simulink model "OPTIM"  (Simulink 4.00)
settings: Solver=ode45  StartTime=0.0  StopTime=40  RelTol=1e-3
settings Model: BlockReductionOpt=off

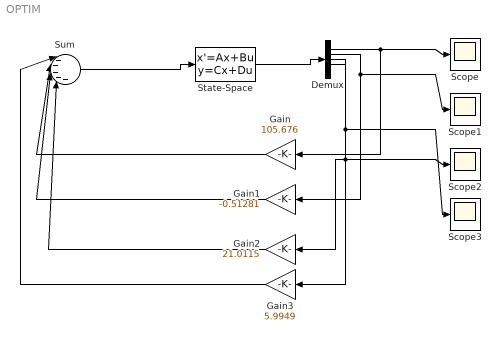
== system OPTIM ==
  Demux : Demux  Outputs=5  BusSelectionMode=off
  Gain : Gain  Orientation=left  Gain=105.676  Multiplication=Element-wise(K.*u)  SaturateOnIntegerOverflow=on
  Gain1 : Gain  Orientation=left  Gain=-0.51281  Multiplication=Element-wise(K.*u)  SaturateOnIntegerOverflow=on
  Gain2 : Gain  Orientation=left  Gain=21.0115  Multiplication=Element-wise(K.*u)  SaturateOnIntegerOverflow=on
  Gain3 : Gain  Orientation=left  Gain=5.9949  Multiplication=Element-wise(K.*u)  SaturateOnIntegerOverflow=on
  Scope{,1..3} (4 alike) : Scope
      Scope settings: TimeRange=auto  YMin=-10  YMax=10  SaveToWorkspace=off  SaveName=ScopeData  LimitDataPoints=on  MaxDataPoints=500000
      Scope1 settings: TimeRange=auto  YMin=-5  YMax=5  SaveToWorkspace=off  LimitDataPoints=on  MaxDataPoints=500000
      Scope2 settings: TimeRange=auto  YMin=-150  YMax=125  SaveToWorkspace=off  SaveName=ScopeData2  LimitDataPoints=on  MaxDataPoints=500000
      Scope3 settings: TimeRange=auto  YMin=-75  YMax=75  SaveToWorkspace=off  SaveName=ScopeData3  LimitDataPoints=on  MaxDataPoints=500000
  State-Space : StateSpace  A=[0 1 0 0 0; 0 -16 -9.8178 0 623.16; 0 0 0 1 0; -8.7478 0.15147 -3.2745 -0.02575 0; 0 -144740 0 0 -475]  B=[0 0 0 0 250]'  C="[1 0 0 0 0  ;0 1 0 0 0 ;0 0 1 0  0;0 0 0 1 0 ;0 0 0 0 1]"  D=[0 0 0 0 0]'  X0=[5 0 30 0 0]  Realization=auto  AbsoluteTolerance=auto
  Sum : Sum  Inputs=|-----  SaturateOnIntegerOverflow=on
  wires:
  State-Space/1 -> Demux/1
  Demux/1 -> Gain/1, Scope/1
  Demux/2 -> Gain1/1, Scope1/1
  Demux/3 -> Gain2/1, Scope2/1
  Demux/4 -> Scope3/1, Gain3/1
  Gain/1 -> Sum/2
  Gain1/1 -> Sum/3
  Gain2/1 -> Sum/4
  Gain3/1 -> Sum/1
  Sum/1 -> State-Space/1
